simulink model "PV_2017a"  (R2017a)
settings: Solver=ode3  StartTime=0.0  StopTime=1.5  FixedStep=5e-6  RelTol=1e-3
libraries: spsSeriesRLCBranchLib x2, spsPVArrayLib x2, spspowerguiLib x1
settings Model: Creator=guler  LastModifiedBy=dudekpob
settings OptimizationCC: LifeSpan=inf
settings DebuggingCC: SFExecutionAtInitializationDiag=none
settings HardwareCC: ProdBitPerSizeT=32  ProdBitPerPtrDiffT=32  ProdWordSize=32  ProdHWDeviceType=Specified
settings SimscapeCC: SimscapeNormalizeSystem=off

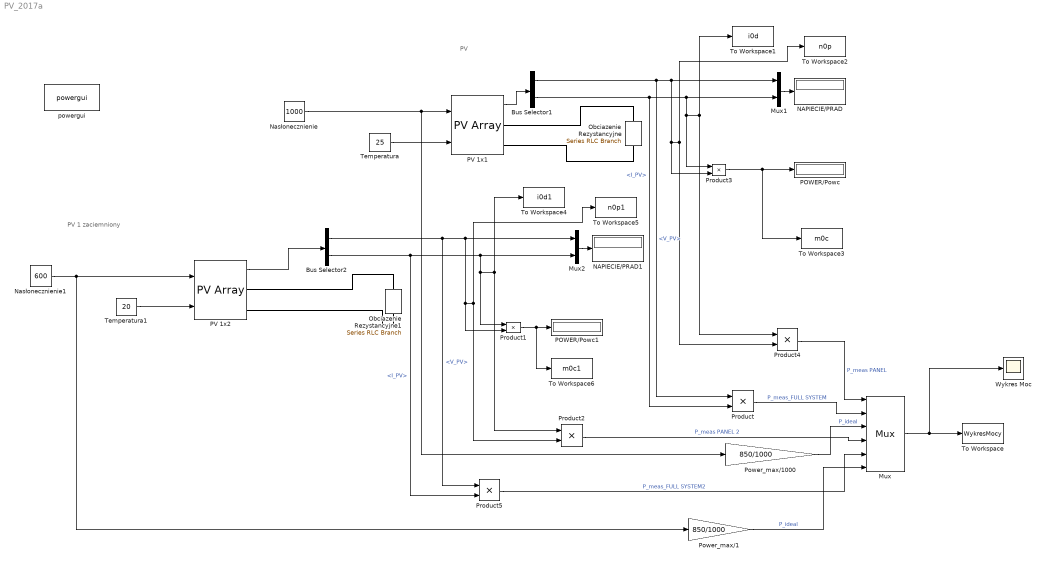
== system PV_2017a ==
  note: PV
  note: PV 1 zaciemniony
  Bus Selector1 : BusSelector  OutputSignals=V_PV,I_PV
  Bus Selector2 : BusSelector  OutputSignals=V_PV,I_PV
  Mux : Mux  Inputs=6
  Mux1 : Mux  Inputs=2
  Mux2 : Mux  Inputs=2
  NAPIECIE/PRAD : Display
  NAPIECIE/PRAD1 : Display
  Nasłonecznienie : Constant  Value=1000
  Nasłonecznienie1 : Constant  Value=600
  Obciazenie Rezystancyjne : spsSeriesRLCBranchLib/Series RLC Branch  LConnTagsString=__new0  RConnTagsString=__new0  BranchType=R  Resistance=12.5  Inductance=1e-3  SetiL0=off  InitialCurrent=0  Capacitance=100e-6  Setx0=off  InitialVoltage=0  Measurements=None
  Obciazenie Rezystancyjne1 : spsSeriesRLCBranchLib/Series RLC Branch  LConnTagsString=__new0  RConnTagsString=__new0  BranchType=R  Resistance=12.5  Inductance=1e-3  SetiL0=off  InitialCurrent=0  Capacitance=100e-6  Setx0=off  InitialVoltage=0  Measurements=None
  POWER/Powc : Display
  POWER/Powc1 : Display
  PV 1x1 : spsPVArrayLib/PV Array  Npar=1  Nser=1  PlotType=array @ 1000 W/m2 & specified temperatures  S_vec="[ 1000  500  300 ]"  Temp_C_vec=[25 40]  ModuleName=User-defined  PlotWhenSelected=off  Pm=213.15  Ncell=60  Voc=36.3  Isc=7.84  Vm=29  Im=7.35  beta_Voc_pc=-0.36099  alpha_Isc_pc=0.102  beta_Voc=-0.13104  alpha_Isc=0.0079968  IL=7.8654  I0=2.9273e-10  nI=0.98119  Rsh=313.0553  Rs=0.39381  RobustModel=off  RobustCellTemperature=313.3991  BAL=off  Tc=1e-6  Tfilter=5e-4
  PV 1x2 : spsPVArrayLib/PV Array  Npar=1  Nser=1  PlotType=array @ 1000 W/m2 & specified temperatures  S_vec="[ 1000  500  300 ]"  Temp_C_vec=[ 25 40]  ModuleName=User-defined  PlotWhenSelected=off  Pm=213.15  Ncell=60  Voc=36.3  Isc=7.84  Vm=29  Im=7.35  beta_Voc_pc=-0.36099  alpha_Isc_pc=0.102  beta_Voc=-0.13104  alpha_Isc=0.0079968  IL=7.8654  I0=2.9273e-10  nI=0.98119  Rsh=313.0553  Rs=0.39381  RobustModel=off  RobustCellTemperature=313.3991  BAL=off  Tc=1e-6  Tfilter=5e-4
  Power_max/1 : Gain  Gain=850/1000
  Power_max/1000 : Gain  Gain=850/1000
  Product{,1..5} (6 alike) : Product
  Temperatura : Constant  Value=25
  Temperatura1 : Constant  Value=20
  To Workspace : ToWorkspace  VariableName=WykresMocy  SaveFormat=Timeseries  SampleTime=-1
  To Workspace1 : ToWorkspace  VariableName=i0d  SaveFormat=Timeseries  SampleTime=-1
  To Workspace2 : ToWorkspace  VariableName=n0p  SaveFormat=Timeseries  SampleTime=-1
  To Workspace3 : ToWorkspace  VariableName=m0c  SaveFormat=Timeseries  SampleTime=-1
  To Workspace4 : ToWorkspace  VariableName=i0d1  SaveFormat=Timeseries  SampleTime=-1
  To Workspace5 : ToWorkspace  VariableName=n0p1  SaveFormat=Timeseries  SampleTime=-1
  To Workspace6 : ToWorkspace  VariableName=m0c1  SaveFormat=Timeseries  SampleTime=-1
  Wykres Moc : Scope
  powergui : spspowerguiLib/powergui  Priority=1  SimulationMode=Discrete  SampleTime=5e-6  frequency=60  Iterations=50  frequencyindice=0  Pbase=100e6  ErrMax=1e-4  UnitsV=kV  UnitsW=MW  buscounter=0  FunctionMessages=off  echomessages=off  EnableUseOfTLC=off  CurrentSourceSwitches=off  DisableSnubberDevices=off  DisableRonSwitches=off  DisableVfSwitches=off  DisplayEquations=off  AutomaticDiscreteSolvers=off  SolverType=Tustin/Backward Euler (TBE)  Interpol=off  ExternalGateDelay=off  methode=off  Ts=100  x0status=blocks  SPID=on  SwTol=0  HookPort=off  NonlinearTolerance=1e-4  nMaxIteration=100  ContinueOnMaxIteration=off  RestoreLinks=warning  ResistiveCurrentMeasurement=off  Frange=[0:2:500]  Ylog=off  Xlog=on  ShowGrid=off  save=off  variable=ZData  structure=0  ZoomFFT=off  StartTime=0.0  cycles=1  DisplayStyle=1  fundamental=60  FreqAxis=off  MaxFrequency=1000  frequencyindicesteady=1  RmsSteady=1  display=off
  wires:
  Product4/1 -> Mux/1  "P_meas PANEL"
  Power_max/1000/1 -> Mux/3  "P_ideal"
  Nasłonecznienie/1 -> Power_max/1000/1, PV 1x1/1
  Mux/1 -> Wykres Moc/1, To Workspace/1
  Product/1 -> Mux/2  "P_meas_FULL SYSTEM"
  Product3/1 -> To Workspace3/1, POWER/Powc/1
  Bus Selector1/1 -> Product/1, Product3/2, Product4/2, To Workspace2/1, Mux1/1  "<V_PV>"
  Mux1/1 -> NAPIECIE/PRAD/1
  Temperatura/1 -> PV 1x1/2
  Bus Selector1/2 -> Product/2, Product3/1, Product4/1, To Workspace1/1, Mux1/2  "<I_PV>"
  PV 1x1/1 -> Bus Selector1/1
  Temperatura1/1 -> PV 1x2/2
  PV 1x2/1 -> Bus Selector2/1
  Bus Selector2/2 -> Product5/2, Mux2/2, Product1/1, Product2/1, To Workspace4/1  "<I_PV>"
  Bus Selector2/1 -> Product5/1, Mux2/1, Product1/2, Product2/2, To Workspace5/1  "<V_PV>"
  Mux2/1 -> NAPIECIE/PRAD1/1
  Product1/1 -> To Workspace6/1, POWER/Powc1/1
  Product2/1 -> Mux/4  "P_meas PANEL 2"
  Product5/1 -> Mux/5  "P_meas_FULL SYSTEM2"
  Nasłonecznienie1/1 -> Power_max/1/1, PV 1x2/1
  Power_max/1/1 -> Mux/6  "P_ideal"
  connections:
  PV 1x1/RConn2 -- Obciazenie Rezystancyjne/RConn1
  PV 1x1/RConn1 -- Obciazenie Rezystancyjne/LConn1
  PV 1x2/RConn1 -- Obciazenie Rezystancyjne1/LConn1
  PV 1x2/RConn2 -- Obciazenie Rezystancyjne1/RConn1
